simulink model "flight2"  (R2014b)
settings: Solver=ode3  StartTime=0.0  StopTime=10.0  FixedStep=.001  MaxStep=ts_max  RelTol=1e-3  AbsTol=1e-3
values from neighbouring files (symbols this model uses):
  flights = ySspeed(end)    [hopper.m]
  flighty = yS(end)    [hopper.m]
settings Model: Creator=hamidreza  LastModifiedBy=hamidreza

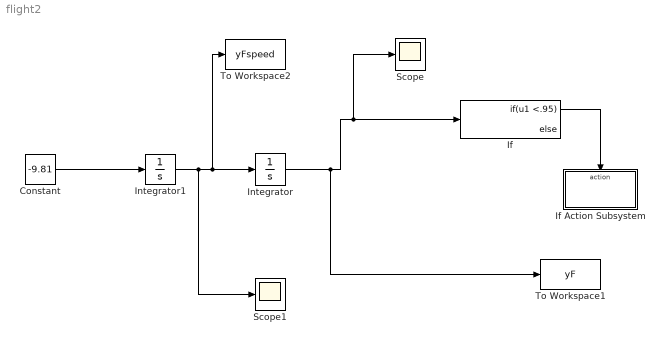
== system flight2 ==
  Constant : Constant  Value=-9.81
  If : If  IfExpression=u1 <.95
  If Action Subsystem : Subsystem  TreatAsAtomicUnit=on
  Integrator : Integrator  InitialCondition=flighty  ZeroCross=off
  Integrator1 : Integrator  InitialCondition=flights
  Scope : Scope
  Scope1 : Scope
  To Workspace1 : ToWorkspace  VariableName=yF  SaveFormat=Structure With Time  SampleTime=-1
  To Workspace2 : ToWorkspace  VariableName=yFspeed  SaveFormat=Structure With Time  SampleTime=-1
  wires:
  Constant/1 -> Integrator1/1
  Integrator1/1 -> Scope1/1, To Workspace2/1, Integrator/1
  If/1 -> If Action Subsystem/Action
  Integrator/1 -> To Workspace1/1, Scope/1, If/1

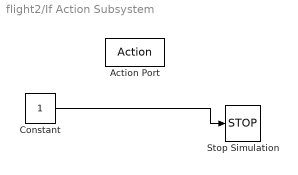
== system flight2/If Action Subsystem ==
  Action Port : ActionPort  ActionType=then
  Constant : Constant
  Stop Simulation : Stop
  wires:
  Constant/1 -> Stop Simulation/1
